simulink model "rev1BB"  (R2021a)
settings: Solver=FixedStepAuto  StartTime=0.0  StopTime=((((preLen+100+dataLenSymbols)*1+pad_first*3)*basePer))*2.5  RelTol=1e-3
values from neighbouring files (symbols this model uses):
  agcDesired = 0    [rev1BB_setup.m]
  agcStep = 2^-8    (= 0.00390625)    [rev1BB_setup.m]
  awgnSeed = abs(dBSnrRange(dBSnrInd)*1000+trial+10000000)    [plotBer.m]    (also in plotBerParSim.m; rev1BB_startup.m = 67)
  basePer = 1/baseFreq    (= 5e-08)    [rev1BB_setup.m]
  bitsPerSymbolHeader = log2(radixHeader)    [rev1BB_setup.m]
  bitsPerSymbolMax = log2(radixMax)    [rev1BB_setup.m]
  cefEarlyWarning = 256    [rev1BB_setup.m]
  cefLen = length(x_CEF)    [rev1BB_setup.m]
  cfoNcoWordLen = 16    [rev1BB_setup.m]
  channelFIR = zeros(1, round(maxSampleDelay)+1)    [rev1BB_simParams_setup.m]
  corr_peak_exclude_trigger = 1+corr_peak_trigger    (= 1.4)    [rev1BB_setup.m]
  corr_peak_trigger = 0.40    (= 0.4)    [rev1BB_setup.m]
  cr_i = 0.020    (= 0.02)    [rev1BB_setup.m]
  cr_i_preamp = 2^-9    (= 0.001953125)    [rev1BB_setup.m]
  cr_p = 0.015    [rev1BB_setup.m]
  dataLenSymbols = header_len_bytes*8/bitsPerSymbolHeader + frame_len_bytes*8/bitsPerSymbol    [rev1BB_setup.m]
  enableTRFreqCorrection = true    [rev1BB_setup.m]
  freeze_agc_in_CEF = true    [rev1BB_setup.m]
  freeze_agc_in_HeaderPayload = true    [rev1BB_setup.m]
  freeze_fineCFO_in_CEF = false    [rev1BB_setup.m]
  freeze_fineCFO_in_HeaderPayload = false    [rev1BB_setup.m]
  golay_type = golayType    (= 32)    [rev1BB_setup.m]
  golayType = 32    [rev1BB_setup.m]
  lmsEqDepth = 16    [rev1BB_setup.m]
  lmsStep_meta = (lmsStep_final - lmsStep_init)/cefLen    [rev1BB_setup.m]
  manChan = false    [rev1BB_simParams_setup.m]
  minSTFPeaks = 3    [rev1BB_setup.m]
  modBPS = [1, 2, 4]    [rev1BB_setup.m]
  modKeys = [0, 1, 2]    [rev1BB_setup.m]
  overSample = 3    [berCurve.m]    (also in rev1BB_setup.m = 4)
  qam16_demod_scale_factor = qam16_hdl_distance/qam16_power_normalized_distance    [rev1BB_setup.m]
  rcRxFilt = rcSqrtFilt    [rev1BB_setup.m]
  rcTxFilt = rcSqrtFilt    [rev1BB_setup.m]
  RxAGCCorrectionLoopPartition = 3    [rev1BB_setup.m]
  RxAGCPwrAvgPartition = 2    [rev1BB_setup.m]
  RxCoarseCFOPartition = 13    [rev1BB_setup.m]
  RxDemodPartition = 15    [rev1BB_setup.m]
  RxEQPartition = 14    [rev1BB_setup.m]
  RxFeedbackPipelining = 64*16    (= 1024)    [rev1BB_setup.m]
  RxFineCFOPartition = 15    [rev1BB_setup.m]
  RxFreezeControllerPartition = 17    [rev1BB_setup.m]
  RxFreezeFeedbackPipelining = RxFeedbackPipelining    (= 1024)    [rev1BB_setup.m]
  RxHeaderDemodPartition = 15    [rev1BB_setup.m]
  RxHeaderParsePartition = 15    [rev1BB_setup.m]
  RxPackerPartition = 16    [rev1BB_setup.m]
  RxPacketControllerPartition = 17    [rev1BB_setup.m]
  RxRRCPartition = 1    [rev1BB_setup.m]
  RxTimingRecoveryControlPartition = 8    [rev1BB_setup.m]
  RxTimingRecoveryDelayAccumPartition = 10    [rev1BB_setup.m]
  RxTimingRecoveryEarlyLatePartition = 10    [rev1BB_setup.m]
  RxTimingRecoveryFreqEstPartition = 10    [rev1BB_setup.m]
  RxTimingRecoveryGolayCorrelatorPartition = 6    [rev1BB_setup.m]
  RxTimingRecoveryGolayPeakDetectPartition = 7    [rev1BB_setup.m]
  RxTimingRecoverySymbolClockPartition = 9    [rev1BB_setup.m]
  RxTimingRecoveryVariableDelayPartition = 5    [rev1BB_setup.m]
  timing_cefEarlyWarningTollerance = 5    [rev1BB_setup.m]
  timing_correlator_pipeline = 1    [rev1BB_setup.m]
  timing_differentiator_grpDelay_roundUp = ceil((timing_differentiator_len)/2+timing_differentiator_pipeline)    [rev1BB_setup.m]
  timing_differentiator_pipeline = 1    [rev1BB_setup.m]
  timing_p = -0.215    [rev1BB_setup.m]
  timing_tolerance = 4    [rev1BB_setup.m]
  timingDifferentiatorFilt = timingDifferentiatorFiltObj.Coefficients    [rev1BB_setup.m]
  timingMaxSymbols = dataLenSymbols + length(x_CEF) + length(x_STF)/x_STFRepCount*2+100    [rev1BB_setup.m]
  timingRecoveryDoneSamplesEarly = floor(RxFeedbackPipelining/overSample) - delayToOutputFromDataFSM-1    [rev1BB_setup.m]
  timingRecoveryFreqCorrectionAvgLen = 32    [rev1BB_setup.m]
  timingRecoveryFreqCorrectionDiscardLastN = 2    [rev1BB_setup.m]
  trEarlyLateIGain = -0.000000050    (= -5e-08)    [rev1BB_setup.m]
  trEarlyLatePGain = -0.00225    [rev1BB_setup.m]
  trFarrowTaps = 4    [rev1BB_setup.m]
  trFeedbackPipelining = 64*8    (= 512)    [rev1BB_setup.m]
  trIntPhaseCounterInit = mod(timing_differentiator_grpDelay_roundUp, overSample)    [rev1BB_setup.m]
  trMatch = mod(-trLenToFSM, overSample)    [rev1BB_setup.m]
  trTappedDelayLen = trTappedDelayBase+trFarrowTaps    (= 44)    [rev1BB_setup.m]
  tx_rx_gain = 1    [rev1BB_simParams_setup.m]
  TxResampleModulatorPartition = 1    [rev1BB_setup.m]
  TxRRCFilterPartition = 2    [rev1BB_setup.m]
  txTimingOffset = 0    [plotBer.m]    (also in plotBerParSim.m; rev1BB_startup.m = 2e-05)
  txTimingPhase = channelizerUpDownSampling*overSample*4+1    [rev1BB_simParams_setup.m]
  x_CEF = xSpectrum_CEF_short    [rev1BB_setup.m]
  x_STFRepCount = nSpectrum_STFRepCount_short    (= 60)    [rev1BB_setup.m]
undefined symbols (not defined in the file or in its folder): doppler, magnitude
libraries: simulink x29, rev1CyclopsLib x20, commdigbbndpm3 x9, dspsigops x6, commdigbbndam3 x4, hdlsllib x2, commchan3 x2, commrflib2 x1
(part 3 of 3)

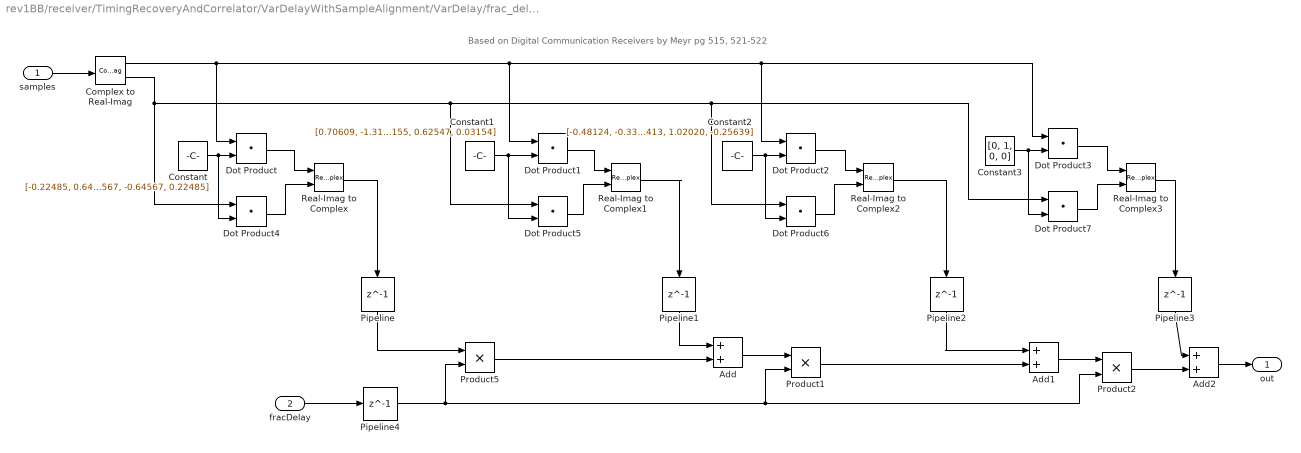
== system rev1BB/receiver/TimingRecoveryAndCorrelator/VarDelayWithSampleAlignment/VarDelay/frac_delay_farrow_N-2_M-3_extState ==
  note: Based on Digital Communication Receivers by Meyr pg 515, 521-522
  samples : Inport  PortDimensions=4
  fracDelay : Inport  Port=2
  Add : Sum
  Add1 : Sum
  Add2 : Sum
  Complex to Real-Imag : ComplexToRealImag
  Constant : Constant  Value=[-0.22485, 0.64567, -0.64567, 0.22485]  OutDataTypeStr=Inherit: Inherit via back propagation
  Constant1 : Constant  Value=[0.70609, -1.31155, 0.62547, 0.03154]  OutDataTypeStr=Inherit: Inherit via back propagation
  Constant2 : Constant  Value=[-0.48124, -0.33413, 1.02020, -0.25639]  OutDataTypeStr=Inherit: Inherit via back propagation
  Constant3 : Constant  Value=[0, 1, 0, 0]  OutDataTypeStr=Inherit: Inherit via back propagation
  Dot Product{,1..7} (8 alike) : DotProduct  InputSameDT=on  OutDataTypeStr=Inherit: Inherit via internal rule
  Pipeline{,1..4} (5 alike) : Delay  DelayLength=1
  Product1 : Product  OutDataTypeStr=Inherit: Same as first input
  Product2 : Product  OutDataTypeStr=Inherit: Same as first input
  Product5 : Product  OutDataTypeStr=Inherit: Same as first input
  Real-Imag to Complex{,1..3} (4 alike) : RealImagToComplex
  out : Outport  VectorParamsAs1DForOutWhenUnconnected=off
  wires:
  Product5/1 -> Add/2
  Real-Imag to Complex3/1 -> Pipeline3/1
  Complex to Real-Imag/1 -> Dot Product/1, Dot Product1/1, Dot Product2/1, Dot Product3/1
  Add1/1 -> Product2/1
  Add2/1 -> out/1
  Real-Imag to Complex/1 -> Pipeline/1
  Add/1 -> Product1/1
  Product2/1 -> Add2/2
  Product1/1 -> Add1/2
  fracDelay/1 -> Pipeline4/1
  Constant/1 -> Dot Product4/2, Dot Product/2
  Constant1/1 -> Dot Product1/2, Dot Product5/2
  Constant2/1 -> Dot Product6/2, Dot Product2/2
  samples/1 -> Complex to Real-Imag/1
  Complex to Real-Imag/2 -> Dot Product4/1, Dot Product6/1, Dot Product7/1, Dot Product5/1
  Constant3/1 -> Dot Product7/2, Dot Product3/2
  Dot Product/1 -> Real-Imag to Complex/1
  Dot Product4/1 -> Real-Imag to Complex/2
  Dot Product1/1 -> Real-Imag to Complex1/1
  Dot Product5/1 -> Real-Imag to Complex1/2
  Real-Imag to Complex1/1 -> Pipeline1/1
  Dot Product2/1 -> Real-Imag to Complex2/1
  Dot Product6/1 -> Real-Imag to Complex2/2
  Real-Imag to Complex2/1 -> Pipeline2/1
  Dot Product3/1 -> Real-Imag to Complex3/1
  Dot Product7/1 -> Real-Imag to Complex3/2
  Pipeline/1 -> Product5/1
  Pipeline1/1 -> Add/1
  Pipeline2/1 -> Add1/1
  Pipeline3/1 -> Add2/1
  Pipeline4/1 -> Product5/2, Product1/2, Product2/2

== system rev1BB/receiver/SymbolDomainOuter/VITIS_CLOCK_DOMAIN_SymbolDomain/CoarseCFOCorrect/CoarseCFOEstimate/ComplexConj ==
  In1 : Inport
  Complex to Real-Imag : ComplexToRealImag
  Gain : Gain  Gain=-1
  Real-Imag to Complex : RealImagToComplex
  Out1 : Outport
  wires:
  In1/1 -> Complex to Real-Imag/1
  Real-Imag to Complex/1 -> Out1/1
  Complex to Real-Imag/1 -> Real-Imag to Complex/1
  Complex to Real-Imag/2 -> Gain/1
  Gain/1 -> Real-Imag to Complex/2

== system rev1BB/receiver/SymbolDomainOuter/VITIS_CLOCK_DOMAIN_SymbolDomain/FineCFOCorrect/EstPhase/findNearestConstPt ==
  symbol : Inport
  modulationMode : Inport  Port=2
  BPSK Demodulator Baseband : commdigbbndpm3/BPSK Demodulator Baseband  DecType=Hard decision  VarSource=Dialog  Variance=1  Ph=0  outDtype=uint8  derotateFactorWordLen=16  derotateFactorDataTypeStr=Inherit: Same word length as input  derotateFactorLastDataTypeStr=Inherit: Same word length as input
  BPSK Modulator Baseband : commdigbbndpm3/BPSK Modulator Baseband  Ph=0  outDtype=single  outWordLen=16  outUDDataType=sfix(16)  outFracLenMode=Best precision  outFracLen=15  outDataTypeStr=single  outLastDataTypeStr=single
  Gain : Gain  Gain=qam16_demod_scale_factor
  Multiport Switch : MultiPortSwitch  DataPortOrder=Zero-based contiguous  zeroidx=on
  QPSK Demodulator Baseband : commdigbbndpm3/QPSK Demodulator Baseband  OutType=Integer  DecType=Hard decision  VarSource=Dialog  Variance=1  Dec=Gray  Ph=pi/4  outDtype1=Inherit via internal rule  outDtype2=uint8  derotateFactorWordLen=16  derotateFactorDataTypeStr=Inherit: Same word length as input  derotateFactorLastDataTypeStr=Inherit: Same word length as input
  QPSK Modulator Baseband : commdigbbndpm3/QPSK Modulator Baseband  InType=Integer  Enc=Gray  Ph=pi/4  outDtype=single  outWordLen=16  outUDDataType=sfix(16)  outFracLenMode=Best precision  outFracLen=15  outDataTypeStr=single  outLastDataTypeStr=single
  Rectangular QAM Demodulator Baseband : commdigbbndam3/Rectangular QAM Demodulator Baseband  M=16  OutType=Integer  DecType=Hard decision  VarSource=Dialog  Variance=1  Dec=Gray  Mapping=[0:15]  PowType=Min. distance between symbols  MinDist=qam16_hdl_distance  AvgPow=1  PeakPow=1  Ph=0  outDtype1=Inherit via internal rule  outDtype2=uint8  derotateFactorWordLen=16  derotateFactorDataTypeStr=Inherit: Same word length as input  derotateFactorLastDataTypeStr=Inherit: Same word length as input  denormFactorWordLen=16  denormFactorDataTypeStr=Inherit: Same word length as input  denormFactorLastDataTypeStr=Inherit: Same word length as input  prodOutWordLen=32  prodOutOverflowMode=Wrap  prodOutRoundingMode=Floor  prodOutOvFlMode=off  prodOutOvFlModeLastStrValue=off  sumWordLen=32
  Rectangular QAM Modulator Baseband : commdigbbndam3/Rectangular QAM Modulator Baseband  M=16  InType=Integer  Enc=Gray  Mapping=[0:15]  PowType=Average Power  MinDist=2  AvgPow=1  PeakPow=1  Ph=0  outDtype=single  outWordLen=16  outUDDataType=sfix(16)  outFracLenMode=Best precision  outFracLen=15  outDataTypeStr=single  outLastDataTypeStr=single
  nearestPt : Outport
  wires:
  symbol/1 -> BPSK Demodulator Baseband/1, Gain/1, QPSK Demodulator Baseband/1
  BPSK Demodulator Baseband/1 -> BPSK Modulator Baseband/1
  QPSK Demodulator Baseband/1 -> QPSK Modulator Baseband/1
  Gain/1 -> Rectangular QAM Demodulator Baseband/1
  Rectangular QAM Demodulator Baseband/1 -> Rectangular QAM Modulator Baseband/1
  modulationMode/1 -> Multiport Switch/1
  BPSK Modulator Baseband/1 -> Multiport Switch/2
  QPSK Modulator Baseband/1 -> Multiport Switch/3
  Rectangular QAM Modulator Baseband/1 -> Multiport Switch/4
  Multiport Switch/1 -> nearestPt/1

== system rev1BB/receiver/SymbolDomainOuter/VITIS_CLOCK_DOMAIN_SymbolDomain/FineCFOCorrect/PhaseCorrectionAccumulator/PseudoFMod2Pi ==
  In1 : Inport
  Compare To Constant : simulink/Logic and Bit Operations/Compare To Constant  relop=<  const=-2*pi  OutDataTypeStr=boolean
  Constant1 : Constant  Value=2*pi  OutDataTypeStr=Inherit: Inherit via back propagation
  Constant2 : Constant  Value=2*pi  OutDataTypeStr=Inherit: Inherit via back propagation
  Sum : Sum  Inputs=|+-  OutDataTypeStr=Inherit: Same as first input
  Sum1 : Sum  Inputs=|++  OutDataTypeStr=Inherit: Same as first input
  Switch1 : Switch  Criteria=u2 > Threshold  Threshold=2*pi
  Switch2 : Switch  Criteria=u2 ~= 0  Threshold=2*pi
  Out1 : Outport
  wires:
  Switch2/1 -> Out1/1
  Switch1/1 -> Sum1/1, Switch2/3, Compare To Constant/1
  Sum/1 -> Switch1/1
  Sum1/1 -> Switch2/1
  In1/1 -> Sum/1, Switch1/2, Switch1/3
  Constant1/1 -> Sum/2
  Constant2/1 -> Sum1/2
  Compare To Constant/1 -> Switch2/2

== system rev1BB/receiver/SymbolDomainOuter/VITIS_CLOCK_DOMAIN_SymbolDomain/FineCFOCorrect/PhaseCorrectionAccumulator/Shift180 ==
  correction : Inport
  shift180 : Inport  Port=2
  Sum : Sum  Inputs=++|  OutDataTypeStr=Inherit: Same as first input
  Switch : Switch  Criteria=u2 ~= 0
  pi : Constant  Value=pi
  correctionOut : Outport
  wires:
  correction/1 -> Sum/1, Switch/3
  pi/1 -> Sum/2
  Sum/1 -> Switch/1
  shift180/1 -> Switch/2
  Switch/1 -> correctionOut/1

== stateflow chart rev1BB/receiver/TimingRecoveryAndCorrelator/TRControl/tr_control ==
  settings: executeAtInitialization=1
  note: Because of multipath, multiple peaks
      | may appear close together, do not
      | interpret these as error events
  state Reset
    entry:
    periodCount = int32(0);
    peakCount = int32(0);
    resetIntegerPhase=true;
    receiving=false;
    estimateOK=false;
    estimateNow=false;
    trEstDone=false;
    lastPeriod=int32(0);
  state DummyInit
    entry:
    periodCount = int32(0);
    peakCount = int32(0);
    resetIntegerPhase=true;
    receiving=false;
    estimateOK=false;
    estimateNow=false;
    trEstDone=false;
    lastPeriod=int32(0);
  state BufferFirst
    entry:
    periodCount = int32(1);
    peakCount = int32(1);
    resetIntegerPhase = true;
    receiving=true;
    estimateOK=true;
    estimateNow=true;
    trEstDone=false;
    lastPeriod=int32(golay_type*overSample);
  state WaitForNext
    entry:
    periodCount = periodCount + int32(1);
    resetIntegerPhase = false;
    receiving=true;
    estimateOK=true;
    estimateNow=false;
    trEstDone=false;
  state NextPeak
    entry:
    lastPeriod=periodCount;
    periodCount = int32(1);
    peakCount = peakCount + int32(1);
    resetIntegerPhase = false;
    receiving=true;
    estimateOK=true;
    estimateNow=true;
    trEstDone=false;
  note: Dummy initial state to ensure
      | proper init entry events occur
      | after FSM reset (from init C
      | function)
  note: This came from the packet processor in the symbol domain
  state Hold
    entry:
    resetIntegerPhase = false;
    receiving=true;
    estimateOK=false;
    estimateNow=false;
    trEstDone=true;
    periodCount = periodCount+1;
  (default) -> DummyInit
  Reset -> BufferFirst [order 1] : [peak == true]
  DummyInit -> Reset
  WaitForNext -> NextPeak [order 2] : [periodCount >= golay_type*overSample-timing_tolerance && periodCount <= golay_type*overSample+timing_tolerance && periodCount > overSample && peak == true]
  BufferFirst -> WaitForNext
  Reset -> Reset [order 2] : [peak == false]
  NextPeak -> WaitForNext [order 2]
  WaitForNext -> Reset [order 3] : [periodCount > max(golay_type*overSample+timing_tolerance, golay_type*overSample+timing_cefEarlyWarningTollerance)]
  WaitForNext -> WaitForNext [order 4]
  WaitForNext -> Hold [order 1] : [((periodCount >= golay_type*overSample-timing_cefEarlyWarningTollerance && periodCount <= golay_type*overSample+timing_cefEarlyWarningTollerance && periodCount > overSample) || (periodCount<timing_cefEarlyWarningTollerance)) && peakCount >= minSTFPeaks && peakCount <= (x_STFRepCount+1) && cef_start == true]
  Hold -> Reset [order 2] : [periodCount > timingMaxSymbols*overSample]
  Hold -> Reset [order 1] : [rst == true]
  NextPeak -> Hold [order 1] : [peakCount>=minSTFPeaks && peakCount <= (x_STFRepCount+1) && cef_start == true]
  data: peak input boolean; periodCount local int32; rst input boolean; golay_type parameter int32; resetIntegerPhase output; peakCount local int32; receiving output boolean; overSample parameter int32; minSTFPeaks parameter int32; cef_start input; x_STFRepCount parameter int32; estimateOK output boolean; estimateNow output boolean; timing_tolerance parameter int32; trEstDone output boolean; lastPeriod output int32; timing_cefEarlyWarningTollerance parameter int32; timingMaxSymbols parameter int32

== stateflow chart rev1BB/receiver/SymbolDomainOuter/VITIS_CLOCK_DOMAIN_SymbolDomain/CoarseCFOCorrect/CoarseCFOEstimate/cfo_est_control ==
  settings: executeAtInitialization=1
  state Reset
    entry:
    buffer = false;
    calcDiff = false;
    periodCount = int32(0);
    peakCount = int32(0);
    cur_re = 0.0;
    cur_im = 0.0;
    prev_re = 0.0;
    prev_im = 0.0;
  state BufferFirst
    entry:
    buffer = true;
    cur_re = correlation_re;
    cur_im = correlation_im;
    calcDiff = false;
    periodCount = int32(1);
  state WaitForNext
    entry:
    buffer = false;
    calcDiff = false;
    periodCount = periodCount + int32(1);
  state CalculateDiff
    entry:
    buffer = true;
    prev_re = cur_re;
    prev_im = cur_im;
    cur_re = correlation_re;
    cur_im = correlation_im;
    calcDiff = true;
    peakCount = peakCount + int32(1);
    periodCount = int32(1);
  state DummyInit
    entry:
    buffer = false;
    calcDiff = false;
    periodCount = int32(0);
    peakCount = int32(0);
  note: Dummy initial state to ensure
      | proper init entry events occur
      | after FSM reset (from init C
      | function)
  state HoldDiff
    entry:
    buffer = false;
    calcDiff = false;
  CalculateDiff -> Reset [order 1] : [rst == true]
  WaitForNext -> Reset [order 1] : [rst == true]
  CalculateDiff -> WaitForNext [order 3]
  BufferFirst -> Reset [order 1] : [rst == true]
  (default) -> DummyInit
  Reset -> BufferFirst [order 1] : [peak == true]
  BufferFirst -> WaitForNext [order 3]
  DummyInit -> Reset
  WaitForNext -> CalculateDiff [order 3] : [periodCount >= golay_type ]
  Reset -> Reset [order 2] : [peak == false]
  WaitForNext -> WaitForNext [order 4]
  WaitForNext -> HoldDiff [order 2] : [stop == true]
  BufferFirst -> HoldDiff [order 2] : [stop == true]
  HoldDiff -> Reset : [rst == true]
  CalculateDiff -> HoldDiff [order 2] : [stop == true]
  data: cur_re output single; cur_im output single; peak input boolean; correlation_re input; correlation_im input; prev_re output single; prev_im output single; calcDiff output boolean; periodCount local int32; stop input boolean; rst input boolean; peakCount output int32; buffer output boolean; golay_type parameter int32

== stateflow chart rev1BB/receiver/SymbolDomainOuter/VITIS_CLOCK_DOMAIN_SymbolDomain/HeaderParser/header_parse ==
  settings: executeAtInitialization=1
  state ParseLen
    entry:
    len = bitor(bitsrl(len, bitsPerSymbolHeader), bitsll(uint16(data), 16-bitsPerSymbolHeader));
    counter = counter + uint8(bitsPerSymbolHeader);
  state Hold
    entry:
    payload = true;
    payload_early=true;
    done_parsing = true;
  state ParseNet_Id
    entry:
    net_id = bitor(bitsrl(len, bitsPerSymbolHeader), bitsll(uint16(data), 16-bitsPerSymbolHeader));
    counter = counter + uint8(bitsPerSymbolHeader);
  state ParseDst
    entry:
    dst = bitor(bitsrl(dst, bitsPerSymbolHeader), bitsll(data, 8-bitsPerSymbolHeader));
    counter = counter + uint8(bitsPerSymbolHeader);
  state ParseSrc
    entry:
    src = bitor(bitsrl(src, bitsPerSymbolHeader), bitsll(data, 8-bitsPerSymbolHeader));
    counter = counter + uint8(bitsPerSymbolHeader);
  state ParseModType
    entry:
    mod_type = bitor(bitsrl(mod_type, bitsPerSymbolHeader),bitsll(data, 8-bitsPerSymbolHeader));
    counter = counter + uint8(bitsPerSymbolHeader);
  state Waiting
    entry:
    counter = uint8(0);
    mod_type = uint8(0);
    mod_type_valid = false;
    type = uint8(0);
    type_valid = false;
    src = uint8(0);
    src_valid = false;
    dst = uint8(0);
    dst_valid = false;
    net_id = uint16(0);
    net_id_valid = false;
    len = uint16(0);
    len_valid = false;
    done_parsing = false;
    payload = false;
    payload_early=false;
  state ParseType
    entry:
    type = bitor(bitsrl(type, bitsPerSymbolHeader),bitsll(data, 8-bitsPerSymbolHeader));
    counter = counter + uint8(bitsPerSymbolHeader);
  state DummyInit
    entry:
    counter = uint8(0);
    mod_type = uint8(0);
    mod_type_valid = false;
    type = uint8(0);
    type_valid = false;
    src = uint8(0);
    src_valid = false;
    dst = uint8(0);
    dst_valid = false;
    net_id = uint16(0);
    net_id_valid = false;
    len = uint16(0);
    len_valid = false;
    done_parsing = false;
    payload = false;
    payload_early=false;
  state ParseLenLast
    entry:
    len = bitor(bitsrl(len, bitsPerSymbolHeader), bitsll(uint16(data), 16-bitsPerSymbolHeader));
    len_valid = true;
    payload_early=true;
    counter = uint8(0);
  state ParseModTypeLast
    entry:
    mod_type = bitor(bitsrl(mod_type, bitsPerSymbolHeader), bitsll(data, 8-bitsPerSymbolHeader));
    mod_type_valid = true;
    counter = uint8(0);
  state ParseTypeLast
    entry:
    type = bitor(bitsrl(type, bitsPerSymbolHeader), bitsll(data, 8-bitsPerSymbolHeader));
    type_valid = true;
    counter = uint8(0);
  state ParseNet_IdLast
    entry:
    net_id = bitor(bitsrl(len, bitsPerSymbolHeader), bitsll(uint16(data), 16-bitsPerSymbolHeader));
    net_id_valid = true;
    counter = uint8(0);
  state ParseSrcLast
    entry:
    src = bitor(bitsrl(src, bitsPerSymbolHeader), bitsll(data, 8-bitsPerSymbolHeader));
    src_valid = true;
    counter = uint8(0);
  state ParseDstLast
    entry:
    dst = bitor(bitsrl(dst, bitsPerSymbolHeader), bitsll(data, 8-bitsPerSymbolHeader));
    dst_valid = true;
    counter = uint8(0);
  ParseLenLast -> Waiting [order 1] : [rst==true]
  ParseNet_IdLast -> Waiting [order 1] : [rst==true]
  ParseNet_Id -> Waiting [order 1] : [rst==true]
  ParseLen -> Waiting [order 1] : [rst==true]
  ParseDstLast -> Waiting [order 1] : [rst==true]
  ParseDst -> Waiting [order 1] : [rst==true]
  ParseSrcLast -> Waiting [order 1] : [rst==true]
  ParseSrc -> Waiting [order 1] : [rst==true]
  ParseTypeLast -> Waiting [order 1] : [rst==true]
  ParseType -> Waiting [order 1] : [rst==true]
  ParseModTypeLast -> Waiting [order 1] : [rst==true]
  ParseLen -> ParseLen [order 3] : [counter < 16-bitsPerSymbolHeader ]
  Hold -> Hold [order 2]
  ParseNet_Id -> ParseNet_Id [order 3] : [counter < 16-bitsPerSymbolHeader ]
  ParseModType -> Waiting [order 2] : [rst==true]
  ParseDst -> ParseDst [order 3] : [counter < 8-bitsPerSymbolHeader ]
  ParseSrc -> ParseSrc [order 3] : [counter < 8-bitsPerSymbolHeader ]
  ParseModType -> ParseModType [order 3] : [counter < 8-bitsPerSymbolHeader ]
  ParseType -> ParseType [order 3] : [counter < 8-bitsPerSymbolHeader ]
  ParseNet_IdLast -> ParseLen [order 2]
  ParseLen -> ParseLenLast [order 2] : [counter >= 16-bitsPerSymbolHeader ]
  (default) -> DummyInit
  ParseLenLast -> Hold [order 2]
  ParseDstLast -> ParseNet_Id [order 2]
  ParseNet_Id -> ParseNet_IdLast [order 2] : [counter >= 16-bitsPerSymbolHeader ]
  Waiting -> ParseModType [order 1] : [valid==true]
  Hold -> Waiting [order 1] : [rst == true]
  ParseModTypeLast -> ParseType [order 2]
  ParseType -> ParseTypeLast [order 2] : [counter >= 8-bitsPerSymbolHeader ]
  ParseModType -> ParseModTypeLast [order 1] : [counter >= 8-bitsPerSymbolHeader ]
  ParseTypeLast -> ParseSrc [order 2]
  ParseSrc -> ParseSrcLast [order 2] : [counter >= 8-bitsPerSymbolHeader ]
  ParseSrcLast -> ParseDst [order 2]
  ParseDst -> ParseDstLast [order 2] : [counter >= 8-bitsPerSymbolHeader ]
  DummyInit -> Waiting
  Waiting -> Waiting [order 2] : [valid==false]
  data: mod_type_valid output boolean; data input uint8; valid input boolean; type_valid output boolean; src_valid output boolean; dst_valid output boolean; len_valid output boolean; done_parsing output boolean; mod_type output uint8; counter local; type output uint8; src output uint8; dst output uint8; len output uint16; rst input boolean; bitsPerSymbolHeader parameter int8; payload output boolean; payload_early output boolean; net_id_valid output boolean; net_id output uint16

== stateflow chart rev1BB/receiver/SymbolDomainOuter/VITIS_CLOCK_DOMAIN_SymbolDomain/DataPacker/dataPacker ==
  settings: executeAtInitialization=1
  state Exe
    note: Used if Max Modulation Scheme is BPSK
    note: Note: It is assumed that the header will exactly fit into the packed representation with no padding required. This simplifies this decoder.
    state HeaderPassThrough
      entry:
      packed_data = data;
      counter = uint8(0);
      valid = true;
      decoding=true;
    state PayloadPassThrough
      entry:
      packed_data = data;
      counter = uint8(0);
      valid = true;
    state PayloadPassThroughLast
      entry:
      packed_data = data;
      counter = uint8(0);
      valid = true;
      last_out=true;
    state FillHeaderOutput
      entry:
      packed_data = bitor(bitsrl(packed_data, bitsPerSymbolHeader),bitsll(data, bitsPerSymbolMax-bitsPerSymbolHeader));
      counter = counter + uint8(bitsPerSymbolHeader);
      valid = true;
      decoding=true;
    state FillPayloadOutput
      entry:
      packed_data = bitor(bitsrl(packed_data, bitsPerSymbolMod),bitsll(data, bitsPerSymbolMax-bitsPerSymbolMod));
      counter = counter + uint8(bitsPerSymbolMod);
      valid = true;
    state FillHeaderFirst
      entry:
      packed_data = bitsll(data, bitsPerSymbolMax-bitsPerSymbolHeader);
      counter = uint8(bitsPerSymbolHeader);
      valid = false;
    state FillHeaderMid
      entry:
      packed_data = bitor(bitsrl(packed_data, bitsPerSymbolHeader),bitsll(data, bitsPerSymbolMax-bitsPerSymbolHeader));
      counter = counter + uint8(bitsPerSymbolHeader);
      valid = false;
    state FillPayloadFirst
      entry:
      packed_data = bitsll(data, bitsPerSymbolMax-bitsPerSymbolMod);
      counter = uint8(bitsPerSymbolMod);
      valid = false;
    state FillPayloadMid
      entry:
      packed_data = bitor(bitsrl(packed_data, bitsPerSymbolMod),bitsll(data, bitsPerSymbolMax-bitsPerSymbolMod));
      counter = counter + uint8(bitsPerSymbolMod);
      valid = false;
    state FillPayloadOutputLast
      entry:
      packed_data = bitor(bitsrl(packed_data, bitsPerSymbolMod),bitsll(data, bitsPerSymbolMax-bitsPerSymbolMod));
      counter = counter + uint8(bitsPerSymbolMod);
      valid = true;
      last_out = true;
    state Err
      entry:
      last_out=true;
      err = true;
    HeaderPassThrough -> HeaderPassThrough [order 3]
    PayloadPassThrough -> PayloadPassThrough [order 2]
    HeaderPassThrough -> PayloadPassThrough [order 1] : [payload == true && bitsPerSymbolMod == bitsPerSymbolMax]
    PayloadPassThrough -> PayloadPassThroughLast [order 1] : [last_in==true]
    FillHeaderOutput -> PayloadPassThrough [order 2] : [payload == true && bitsPerSymbolMod == bitsPerSymbolMax]
    HeaderPassThrough -> FillPayloadFirst [order 2] : [payload == true && bitsPerSymbolMod ~= bitsPerSymbolMax]
    FillHeaderMid -> FillHeaderMid [order 2]
    FillPayloadMid -> FillPayloadMid [order 4]
    FillHeaderFirst -> FillHeaderMid [order 2]
    FillPayloadFirst -> FillPayloadMid [order 3]
    FillHeaderMid -> FillHeaderOutput [order 1] : [counter >=bitsPerSymbolMax-bitsPerSymbolHeader ]
    FillHeaderOutput -> FillPayloadFirst [order 1] : [payload == true && bitsPerSymbolMod ~= bitsPerSymbolMax]
    FillPayloadMid -> FillPayloadOutput [order 1] : [counter >=bitsPerSymbolMax-bitsPerSymbolMod && last_in ==false ]
    FillPayloadMid -> FillPayloadOutputLast [order 2] : [counter >=bitsPerSymbolMax-bitsPerSymbolMod && last_in ==true ]
    FillPayloadOutput -> Err [order 1] : [last_in ==true]
    FillHeaderOutput -> FillHeaderFirst [order 3]
    FillHeaderFirst -> FillHeaderOutput [order 1] : [counter >=bitsPerSymbolMax-bitsPerSymbolHeader ]
    FillPayloadFirst -> FillPayloadOutputLast [order 2] : [last_in ==true]
    FillPayloadOutput -> FillPayloadFirst [order 2]
    FillPayloadFirst -> FillPayloadOutput [order 1] : [counter >=bitsPerSymbolMax-bitsPerSymbolMod && last_in ==false ]
    FillPayloadMid -> Err [order 3] : [counter < bitsPerSymbolMax-bitsPerSymbolMod && last_in ==true ]
  state Waiting
    entry:
    counter = uint8(0);
    packed_data = uint8(0);
    valid = false;
    last_out=false;
    decoding=false;
    err=false;
  state DummyInit
    entry:
    counter = uint8(0);
    packed_data = uint8(0);
    valid = false;
    last_out=false;
    decoding=false;
    err=false;
  PayloadPassThroughLast -> Waiting
  Exe -> Waiting : [rst == true]
  Waiting -> HeaderPassThrough [order 2] : [header==true && bitsPerSymbolMax == 1]
  (default) -> DummyInit
  DummyInit -> Waiting
  Waiting -> FillHeaderFirst [order 1] : [header==true && bitsPerSymbolMax ~= 1]
  Err -> Waiting
  FillPayloadOutputLast -> Waiting
  data: last_in input boolean; header input boolean; bitsPerSymbolMax parameter uint8; bitsPerSymbolMod input uint8; last_out output boolean; packed_data output uint8; bitsPerSymbolHeader parameter uint8; data input uint8; payload input boolean; rst input boolean; valid output boolean; counter local; decoding output boolean; err output boolean

== stateflow chart rev1BB/receiver/SymbolDomainOuter/VITIS_CLOCK_DOMAIN_SymbolDomain/PacketRxController/PreambleTrackingFSM ==
  settings: executeAtInitialization=1
  state Error
    entry:
    err = true;
    waiting = false;
  state STFFirst
    entry:
    stf = true;
    cef_first = false;
    cef = false;
    cef_early = false;
    data = false;
    err = false;
    waiting = false;
    stfCount = 1;
    stfPeaks = stfPeaks + 1;
  state STF
    entry:
    stf = true;
    cef_first = false;
    cef = false;
    cef_early = false;
    data = false;
    err = false;
    waiting = false;
    stfCount = stfCount+1;
  state DummyInit
    entry:
    stf = false;
    cef_first = false;
    cef = false;
    cef_early = false;
    data = false;
    err = false;
    waiting = true;
    stfCount = int32(0);
    stfPeaks = int32(0);
    cefCount = int32(0);
  state Waiting
    entry:
    stf = false;
    cef_first = false;
    cef = false;
    cef_early = false;
    data = false;
    err = false;
    waiting = true;
    stfCount = int32(0);
    stfPeaks = int32(0);
    cefCount = int32(0);
  state CEF_Early_Warning
    entry:
    stf = false;
    cef_first = false;
    cef = true;
    cef_early = true;
    data = false;
    err = false;
    waiting = false;
    cefCount = cefCount +1;
  state CEF_Decision
    entry:
    stf = false;
    cef_first = true;
    cef = true;
    cef_early = false;
    data = false;
    err = false;
    waiting = false;
    cefCount = cefCount +1;
  state CEF
    entry:
    stf = false;
    cef_first = false;
    cef = true;
    cef_early = false;
    data = false;
    err = false;
    waiting = false;
    cefCount = cefCount +1;
  state LastSym
    entry:
    stf = false;
    cef_first = false;
    cef = false;
    cef_early = false;
    data = true;
    err = false;
    waiting = false;
  CEF_Decision -> Error [order 3] : [cefCount >= golay_type && ((cef_start == true))]
  CEF_Decision -> Error [order 2] : [cefCount >= golay_type && ((stf_start == false && cef_start == false))]
  STF -> Error [order 1] : [stfCount >= golay_type && (stf_start==false && cef_start == false) || (stf_start==true && cef_start == true) || (cef_start == true && (stfPeaks < minSTFPeaks || stfPeaks > (x_STFRepCount+1)))]
  Error -> Waiting
  (default) -> DummyInit
  CEF_Early_Warning -> CEF_Early_Warning [order 2]
  CEF -> CEF [order 2]
  CEF_Decision -> CEF_Decision [order 4]
  STFFirst -> STF
  Waiting -> STFFirst : [stf_start==true]
  STF -> CEF_Decision [order 2] : [stfCount >= golay_type && cef_start == true && stfPeaks >= minSTFPeaks && stfPeaks <= (x_STFRepCount+1) ]
  CEF_Decision -> CEF [order 1] : [cefCount >= golay_type && stf_start == true]
  STF -> STFFirst [order 3] : [stfCount >= golay_type && stf_start==true]
  DummyInit -> Waiting
  STF -> STF [order 4]
  LastSym -> Waiting
  CEF_Early_Warning -> LastSym [order 1] : [cefCount >= cefLen]
  CEF -> CEF_Early_Warning [order 1] : [cefCount >= cefLen-cefEarlyWarning]
  data: stf_start input boolean; cef_start input boolean; data output boolean; err output boolean; stf output boolean; cef output boolean; cefCount output int32; stfCount local int32; cefLen parameter int32; cefEarlyWarning parameter int32; cef_early output boolean; waiting output boolean; golay_type parameter; x_STFRepCount parameter; minSTFPeaks parameter; stfPeaks local; cef_first output boolean

== stateflow chart rev1BB/receiver/SymbolDomainOuter/VITIS_CLOCK_DOMAIN_SymbolDomain/PacketRxController/data_control ==
  settings: executeAtInitialization=1
  note: This is to provide a reset to the front part of the
  state Data
    entry:
    valid = true;
    last = false;
    earlyLast = false;
    dataCount = dataCount + int32(1);
  state EarlyWarningLastSym
    entry:
    valid = true;
    last = false;
    earlyLast = true;
    dataCount = dataCount + int32(1);
  state LastSym
    entry:
    valid = true;
    last = true;
    earlyLast = false;
    dataCount = dataCount + int32(1);
  state Waiting
    entry:
    valid = false;
    last = false;
    earlyLast = false;
    startCount = int32(0);
    dataCount = int32(0);
    waitCount = int32(0);
  state DummyInit
    entry:
    valid = false;
    last = false;
    startCount = int32(0);
    dataCount = int32(0);
    waitCount = int32(0);
  Data -> Data [order 2]
  EarlyWarningLastSym -> EarlyWarningLastSym [order 2]
  (default) -> DummyInit
  Waiting -> Data : [preamble_done == true]
  DummyInit -> Waiting
  LastSym -> Waiting
  Data -> EarlyWarningLastSym [order 1] : [dataCount >= dataLenSymbols-1-timingRecoveryDoneSamplesEarly]
  EarlyWarningLastSym -> LastSym [order 1] : [dataCount >= dataLenSymbols-1]
  data: preamble_done input boolean; valid output boolean; startCount local int32; dataCount local int32; waitCount local int32; dataLenSymbols parameter int32; last output boolean; earlyLast output boolean; timingRecoveryDoneSamplesEarly parameter int32
